simulink model "Mask_Editor_SimulinkMask"  (R2015b)
settings: Solver=VariableStepAuto  StartTime=0.0  StopTime=10.0  RelTol=1e-3
settings Model: Creator=LUBO  LastModifiedBy=LUBO

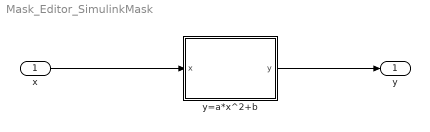
== system Mask_Editor_SimulinkMask ==
  x : Inport
  y=a*x^2+b : Subsystem  mask(Coetom){g_a=2, g_b=2}
      mask prompts: g_a "a"; g_b "b"
      mask help: This demo display how to mask a model
      mask DialogControl g_hyperlink Prompt: Hyo_MATLAB
      mask DialogControl g_hyperlink Callback: web 'http://www.baidu.com'
      mask DialogControl g_pushbutton Prompt: I Love MATLAB!
      mask DialogControl g_pushbutton Callback: web 'http://www.iloveMATLAB.cn/forum.php'
      mask Display: t=0:0.1:10;y=t.^2+1;plot(t,y)
  "y " : Outport
  wires:
  x/1 -> y=a*x^2+b/1(x)
  y=a*x^2+b/1("y ") -> "y "/1

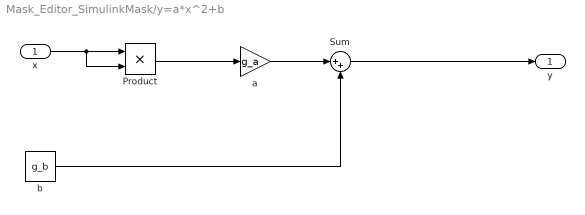
== system Mask_Editor_SimulinkMask/y=a*x^2+b ==
  x : Inport
  Product : Product
  Sum : Sum  Inputs=|++
  a : Gain  Gain=g_a
  b : Constant  Value=g_b
  "y " : Outport
  wires:
  x/1 -> Product/2, Product/1
  b/1 -> Sum/2
  a/1 -> Sum/1
  Sum/1 -> "y "/1
  Product/1 -> a/1
